simulink model "Model"  (R2020a)
settings: Solver=ode3  StartTime=0.0  StopTime=sim.tend  FixedStep=sim.dt  MaxStep=1E-05  RelTol=1e-3
undefined symbols (not defined in the file or in its folder): load
libraries: simulink x11
settings Model: SimulationMode=accelerator  Creator=giai-pron_f  LastModifiedBy=giai-pron_f
settings SolverCC: AlgebraicLoopSolver=LineSearch  AutoInsertRateTranBlk=on  InsertRTBMode=Never (minimum delay)
settings OptimizationCC: DefaultParameterBehavior=Inlined  EnhancedBackFolding=on  PassReuseOutputArgsAs=Individual arguments  ZeroExternalMemoryAtStartup=off  ZeroInternalMemoryAtStartup=off  OptimizeBlockOrder=speed  DifferentSizesBufferReuse=on  EfficientTunableParamExpr=on
settings DebuggingCC: ParameterTunabilityLossMsg=error
settings SFSimCC: MATLABDynamicMemAlloc=off
settings RTWCC: SystemTargetFile=ert.tlc  GenCodeOnly=on  TemplateMakefile=ert_default_tmf  GenerateReport=on  Toolchain=MinGW64 | gmake (64-bit Windows)
settings CodeAppCC: ForceParamTrailComments=on  IgnoreCustomStorageClasses=off  OperatorAnnotations=on  SimulinkDataObjDesc=on  SFDataObjDesc=on  InsertBlockDesc=on
settings ERTTargetCC: TargetLangStandard=C99 (ISO)  GenerateSampleERTMain=on  InlinedParameterPlacement=NonHierarchical  ERTCustomFileTemplate=example_file_process.tlc

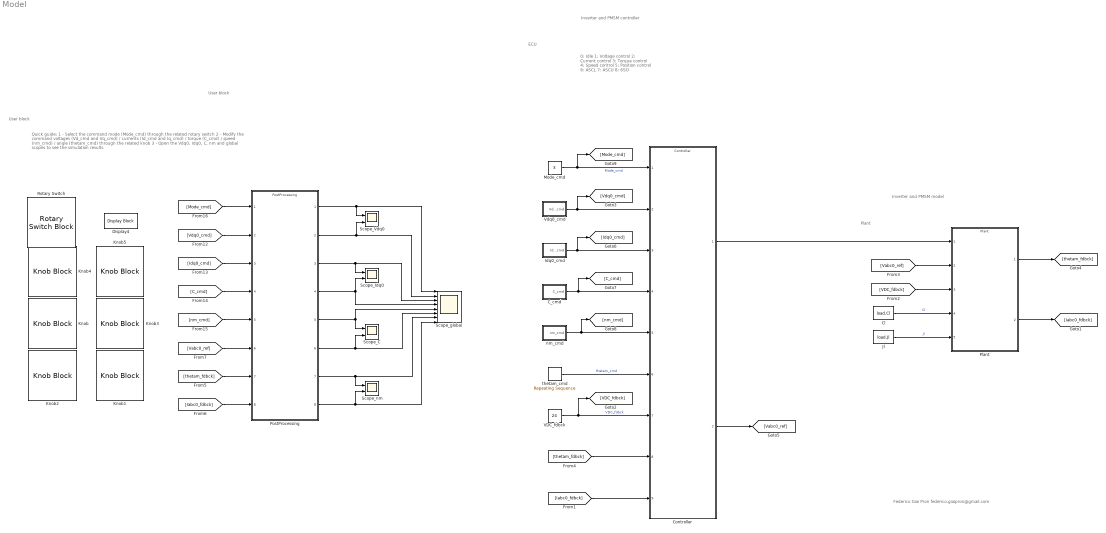
== system Model ==
  note: Quick guide:
      | 1 - Select the command mode (Mode_cmd) through the related rotary switch
      | 2 - Modify the command voltages (Vd_cmd and Vq_cmd) / currents (Id_cmd and Iq_cmd) / torque (C_cmd) / speed (nm_cmd) / angle (thetam_cmd) through the related knob
      | 3 - Open the Vdq0, Idq0, C, nm and global scopes to see the simulation results
  note: Federico Giai Pron
      | federico.giaipron@gmail.com
  note: User block
  note: User block
  note: Plant
  note: ECU
  note: 0: Idle
      | 1: Voltage control
      | 2: Current control
      | 3: Torque control
      | 4: Speed control
      | 5: Position control
      | 6: ASCL
      | 7: ASCU
      | 8: 6SO
  note: Inverter and PMSM controller
  note: Inverter and PMSM model
  C_cmd : Subsystem
  Cl : Constant  Value=load.Cl
  Controller : ModelReference  ModelNameDialog=Controller  ModelReferenceVersion=1.811  CopyOfModelProtected=on
  Display4 : DisplayBlock  LabelPosition=Hide  Format=short  Transparency=1
  Idq0_cmd : Subsystem
  Jl : Constant  Value=load.Jl
  Knob : KnobBlock  ScaleMin=-10  ScaleMax=10
  Knob1 : KnobBlock  ScaleMin=-8000  ScaleMax=8000
  Knob2 : KnobBlock  ScaleMin=-0.3  ScaleMax=0.3
  Knob3 : KnobBlock  ScaleMin=-10  ScaleMax=10
  Knob4 : KnobBlock  ScaleMin=-20  ScaleMax=20
  Knob5 : KnobBlock  ScaleMin=-20  ScaleMax=20
  Mode_cmd : Constant  Value=3
  Plant : ModelReference  ModelNameDialog=Plant  ModelReferenceVersion=1.814  CopyOfModelProtected=on
  PostProcessing : ModelReference  ModelNameDialog=PostProcessing  ModelReferenceVersion=1.816  CopyOfModelProtected=on
  Rotary Switch : RotarySwitchBlock
      settings: Values={{'Idle', 'Voltage', 'Current', 'Torque', 'Speed', 'Position', 'ASCL', 'ASCU', '6SO'}, [0 1 2 3 4 5 6 7 8]}
  Scope_C : Scope  NumInputPorts=2
  Scope_Idq0 : Scope  NumInputPorts=2
  Scope_Vdq0 : Scope  NumInputPorts=2
  Scope_global : Scope  NumInputPorts=8
  Scope_nm : Scope  NumInputPorts=2
  VDC_fdbck : Constant  Value=24
  Vdq0_cmd : Subsystem
  nm_cmd : Subsystem
  thetam_cmd : simulink/Sources/Repeating Sequence  rep_seq_t=[0 0.01 0.011 0.05 0.051 0.1 0.15]  rep_seq_y=0*[0 0 10 10 12 13 30]/10
  wires:
  thetam_cmd/1 -> Controller/6  "thetam_cmd"
  VDC_fdbck/1 -> Controller/7, [VDC_fdbck]  "VDC_fdbck"
  Mode_cmd/1 -> [Mode_cmd], Controller/1  "Mode_cmd"
  Vdq0_cmd/1(Vdq0_cmd) -> [Vdq0_cmd], Controller/2
  [thetam_fdbck] -> Controller/8
  [Iabc0_fdbck] -> Controller/9
  Controller/2 -> [Vabc0_ref]
  [Vabc0_ref] -> Plant/2
  Controller/1 -> Plant/1
  [VDC_fdbck] -> Plant/3
  Cl/1 -> Plant/4  "Cl"
  Jl/1 -> Plant/5  "Jl"
  Plant/1 -> [thetam_fdbck]
  Plant/2 -> [Iabc0_fdbck]
  nm_cmd/1(nm_cmd) -> [nm_cmd], Controller/5
  C_cmd/1(C_cmd) -> [C_cmd], Controller/4
  Idq0_cmd/1(Idq0_cmd) -> [Idq0_cmd], Controller/3
  PostProcessing/6 -> Scope_global/6, Scope_C/2
  PostProcessing/2 -> Scope_Vdq0/2, Scope_global/2
  PostProcessing/7 -> Scope_global/7, Scope_nm/1
  PostProcessing/5 -> Scope_global/5, Scope_C/1
  PostProcessing/3 -> Scope_global/3, Scope_Idq0/1
  PostProcessing/4 -> Scope_Idq0/2, Scope_global/4
  PostProcessing/8 -> Scope_global/8, Scope_nm/2
  PostProcessing/1 -> Scope_global/1, Scope_Vdq0/1
  [Mode_cmd] -> PostProcessing/1
  [Vdq0_cmd] -> PostProcessing/2
  [Idq0_cmd] -> PostProcessing/3
  [C_cmd] -> PostProcessing/4
  [nm_cmd] -> PostProcessing/5
  [Vabc0_ref] -> PostProcessing/6
  [thetam_fdbck] -> PostProcessing/7
  [Iabc0_fdbck] -> PostProcessing/8

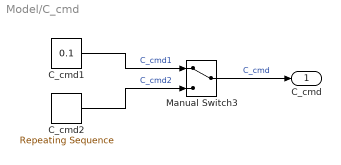
== system Model/C_cmd ==
  C_cmd1 : Constant  Value=0.1
  C_cmd2 : simulink/Sources/Repeating Sequence  rep_seq_t=[0, 0.05, 0.075, 0.125, 0.150, 0.2, 0.25, 0.3]  rep_seq_y=[0, 0, 0.20, 0.20, -0.20, -0.20, 0.1, 0.1]
  Manual Switch3 : ManualSwitch
  C_cmd : Outport
  wires:
  C_cmd1/1 -> Manual Switch3/1  "C_cmd1"
  C_cmd2/1 -> Manual Switch3/2  "C_cmd2"
  Manual Switch3/1 -> C_cmd/1  "C_cmd"

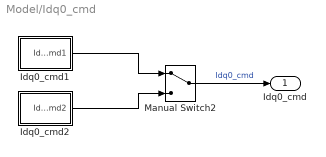
== system Model/Idq0_cmd ==
  Idq0_cmd1 : Subsystem
  Idq0_cmd2 : Subsystem
  Manual Switch2 : ManualSwitch
  Idq0_cmd : Outport
  wires:
  Idq0_cmd1/1(Idq0_cmd1) -> Manual Switch2/1
  Idq0_cmd2/1(Idq0_cmd2) -> Manual Switch2/2
  Manual Switch2/1 -> Idq0_cmd/1  "Idq0_cmd"

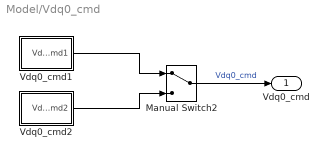
== system Model/Vdq0_cmd ==
  Manual Switch2 : ManualSwitch
  Vdq0_cmd1 : Subsystem
  Vdq0_cmd2 : Subsystem
  Vdq0_cmd : Outport
  wires:
  Vdq0_cmd1/1(Vdq0_cmd1) -> Manual Switch2/1
  Vdq0_cmd2/1(Vdq0_cmd2) -> Manual Switch2/2
  Manual Switch2/1 -> Vdq0_cmd/1  "Vdq0_cmd"

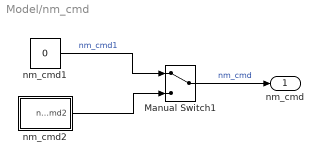
== system Model/nm_cmd ==
  Manual Switch1 : ManualSwitch
  nm_cmd1 : Constant  Value=0
  nm_cmd2 : Subsystem
  nm_cmd : Outport
  wires:
  nm_cmd2/1(nm_cmd2) -> Manual Switch1/2
  Manual Switch1/1 -> nm_cmd/1  "nm_cmd"
  nm_cmd1/1 -> Manual Switch1/1  "nm_cmd1"

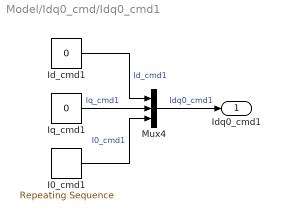
== system Model/Idq0_cmd/Idq0_cmd1 ==
  I0_cmd1 : simulink/Sources/Repeating Sequence  rep_seq_t=[0 100]  rep_seq_y=[0 0]
  Id_cmd1 : Constant  Value=0
  Iq_cmd1 : Constant  Value=0
  Mux4 : Mux  Inputs=3
  Idq0_cmd1 : Outport
  wires:
  Mux4/1 -> Idq0_cmd1/1  "Idq0_cmd1"
  I0_cmd1/1 -> Mux4/3  "I0_cmd1"
  Id_cmd1/1 -> Mux4/1  "Id_cmd1"
  Iq_cmd1/1 -> Mux4/2  "Iq_cmd1"

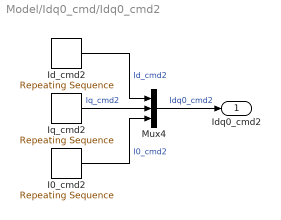
== system Model/Idq0_cmd/Idq0_cmd2 ==
  I0_cmd2 : simulink/Sources/Repeating Sequence  rep_seq_t=[0, 100]  rep_seq_y=[0, 0]
  Id_cmd2 : simulink/Sources/Repeating Sequence  rep_seq_t=[0, 0.1, 0.2, 0.3]  rep_seq_y=[-5, -5, 0, 0]
  Iq_cmd2 : simulink/Sources/Repeating Sequence  rep_seq_t=[0, 0.1, 0.2, 0.3]  rep_seq_y=[0, 0, 5, 5]
  Mux4 : Mux  Inputs=3
  Idq0_cmd2 : Outport
  wires:
  Mux4/1 -> Idq0_cmd2/1  "Idq0_cmd2"
  I0_cmd2/1 -> Mux4/3  "I0_cmd2"
  Id_cmd2/1 -> Mux4/1  "Id_cmd2"
  Iq_cmd2/1 -> Mux4/2  "Iq_cmd2"

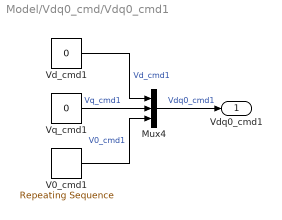
== system Model/Vdq0_cmd/Vdq0_cmd1 ==
  Mux4 : Mux  Inputs=3
  V0_cmd1 : simulink/Sources/Repeating Sequence  rep_seq_t=[0 100]  rep_seq_y=[0 0]
  Vd_cmd1 : Constant  Value=0
  Vq_cmd1 : Constant  Value=0
  Vdq0_cmd1 : Outport
  wires:
  Mux4/1 -> Vdq0_cmd1/1  "Vdq0_cmd1"
  V0_cmd1/1 -> Mux4/3  "V0_cmd1"
  Vd_cmd1/1 -> Mux4/1  "Vd_cmd1"
  Vq_cmd1/1 -> Mux4/2  "Vq_cmd1"

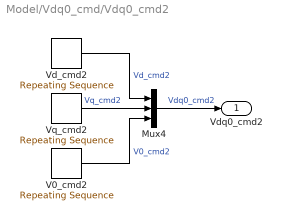
== system Model/Vdq0_cmd/Vdq0_cmd2 ==
  Mux4 : Mux  Inputs=3
  V0_cmd2 : simulink/Sources/Repeating Sequence  rep_seq_t=[0, 100]  rep_seq_y=[0, 0]
  Vd_cmd2 : simulink/Sources/Repeating Sequence  rep_seq_t=[0, 0.1, 0.2, 0.3]  rep_seq_y=[-5, -5, 0, 0]
  Vq_cmd2 : simulink/Sources/Repeating Sequence  rep_seq_t=[0, 0.1, 0.2, 0.3]  rep_seq_y=[0, 0, 5, 5]
  Vdq0_cmd2 : Outport
  wires:
  Mux4/1 -> Vdq0_cmd2/1  "Vdq0_cmd2"
  V0_cmd2/1 -> Mux4/3  "V0_cmd2"
  Vd_cmd2/1 -> Mux4/1  "Vd_cmd2"
  Vq_cmd2/1 -> Mux4/2  "Vq_cmd2"

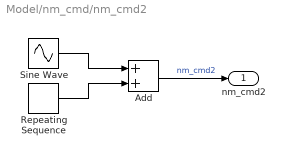
== system Model/nm_cmd/nm_cmd2 ==
  Add : Sum
  Repeating Sequence : simulink/Sources/Repeating Sequence  rep_seq_t=[0, 1, 1.4]  rep_seq_y=[1000 1500 1200]
  Sine Wave : Sin  Amplitude=50  Frequency=5*2*pi  SampleTime=0
  nm_cmd2 : Outport
  wires:
  Repeating Sequence/1 -> Add/2
  Sine Wave/1 -> Add/1
  Add/1 -> nm_cmd2/1  "nm_cmd2"
